simulink library "refrigeration"  (R2014a)
settings: Solver=ode45  StartTime=0.0  StopTime=10.0  RelTol=1e-3
settings Model: Creator=avenger  LastModifiedBy=avenger
settings OptimizationCC: SimCompilerOptimization=off
settings DebuggingCC: MergeDetectMultiDrivingBlocksExec=error  FrameProcessingCompatibilityMsg=error
settings RTWCC: RTWCompilerOptimization=off

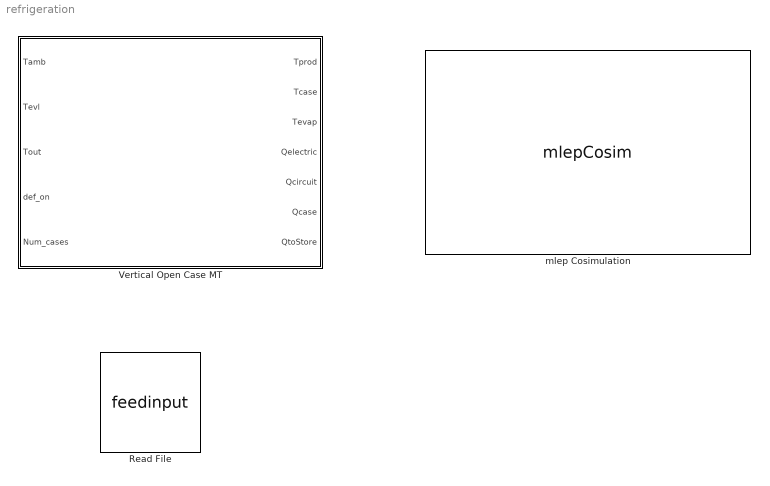
== system refrigeration ==
  Read File : S-Function  FunctionName=feedinput  Parameters=filename,timestep  EnableBusSupport=off  mask(Read Input File){filename='input.txt', timestep=3600}
      mask prompts: filename "File Name:"; timestep "Time Step:"
      mask help:
      | This block reads a file (names passed as parameter) and feeds its input to
      | Simulink at every time step.
  Vertical Open Case MT : Subsystem  AncestorBlock=refrigeration/Vertical Open Case MT
  mlep Cosimulation : S-Function  FunctionName=mlepCosim  Parameters=progname,idf,weather,timeout,step,numinput,numoutput,bcvtbpath  EnableBusSupport=off  mask(S-function: mlepCosim){progname='runenergyplus', idf='supermarket_V810', weather='USA_FL_Miami.Intl.AP.722020_TMY3', timeout=2000, step=300, numinput=1, numoutput=12, bcvtbpath='/home/avenger/Documents/Git/mlep_v2.0/MLE+/bcvtb'}
      mask prompts: progname "E+ Executable:"; idf "IDF File (no .idf extension):"; weather "Weather File (no .epw extension):"; timeout "Timeout (ms):"; step "Sample Time (s):"; numinput "Number of Inputs:"; numoutput "Number of Outputs"; bcvtbpath "Path to bcvtb"
      mask help: This is a S-function block for MLEP.
      mask Display: image('supermarket.png')

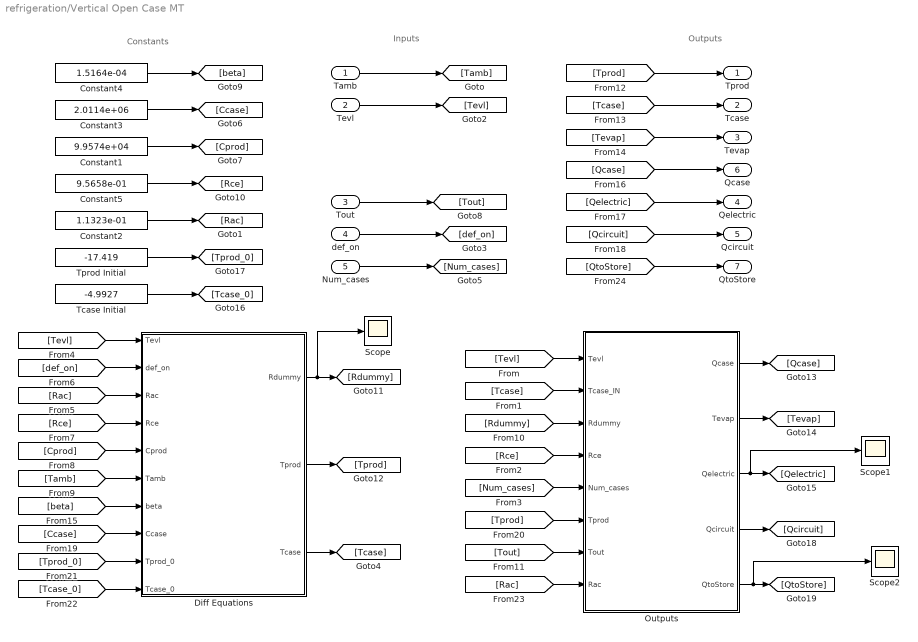
== system refrigeration/Vertical Open Case MT ==
  note: Outputs
  note: Inputs
  note: Constants
  Tamb : Inport
  Tevl : Inport  Port=2
  Tout : Inport  Port=3
  def_on : Inport  Port=4
  Num_cases : Inport  Port=5
  Constant1 : Constant  Value=9.9574e+04
  Constant2 : Constant  Value=1.1323e-01
  Constant3 : Constant  Value=2.0114e+06
  Constant4 : Constant  Value=1.5164e-04
  Constant5 : Constant  Value=9.5658e-01
  Diff Equations : Subsystem
  Outputs : Subsystem
  Scope : Scope
      settings: ShowLegends=on  YMin=-22.5  YMax=32.5
  Scope1 : Scope
      settings: ShowLegends=on  YMin=-22.5  YMax=32.5  SaveName=ScopeData2
  Scope2 : Scope
      settings: ShowLegends=on  YMin=-22.5  YMax=32.5  SaveName=ScopeData7
  Tcase Initial : Constant  Value=-4.9927
  Tprod Initial : Constant  Value=-17.419
  Tprod : Outport
  Tcase : Outport  Port=2
  Tevap : Outport  Port=3
  Qelectric : Outport  Port=4
  Qcircuit : Outport  Port=5
  Qcase : Outport  Port=6
  QtoStore : Outport  Port=7
  wires:
  def_on/1 -> [def_on]
  Num_cases/1 -> [Num_cases]
  Constant3/1 -> [Ccase]
  Constant1/1 -> [Cprod]
  Constant4/1 -> [beta]
  Constant5/1 -> [Rce]
  [Tevl] -> Outputs/1(Tevl)
  [Rce] -> Outputs/4(Rce)
  [Num_cases] -> Outputs/5(Num_cases)
  [Tevl] -> Diff Equations/1(Tevl)
  [Rce] -> Diff Equations/4(Rce)
  [Cprod] -> Diff Equations/5(Cprod)
  [Tamb] -> Diff Equations/6(Tamb)
  Diff Equations/3(Tcase) -> [Tcase]
  Diff Equations/1(Rdummy) -> Scope/1, [Rdummy]
  Diff Equations/2(Tprod) -> [Tprod]
  [Tcase] -> Outputs/2(Tcase_IN)
  [Rdummy] -> Outputs/3(Rdummy)
  [Qelectric] -> Qelectric/1
  [Qcircuit] -> Qcircuit/1
  [Qcase] -> Qcase/1
  Outputs/3(Qelectric) -> Scope1/1, [Qelectric]
  Outputs/1(Qcase) -> [Qcase]
  Outputs/2(Tevap) -> [Tevap]
  Outputs/4(Qcircuit) -> [Qcircuit]
  [beta] -> Diff Equations/7(beta)
  [Ccase] -> Diff Equations/8(Ccase)
  [Tprod] -> Outputs/6(Tprod)
  Tprod Initial/1 -> [Tprod_0]
  Tcase Initial/1 -> [Tcase_0]
  Tamb/1 -> [Tamb]
  Tevl/1 -> [Tevl]
  [Tprod] -> Tprod/1
  [Tcase] -> Tcase/1
  [Tevap] -> Tevap/1
  [Rac] -> Diff Equations/3(Rac)
  [def_on] -> Diff Equations/2(def_on)
  Constant2/1 -> [Rac]
  [Tprod_0] -> Diff Equations/9(Tprod_0)
  [Tcase_0] -> Diff Equations/10(Tcase_0)
  Tout/1 -> [Tout]
  [Tout] -> Outputs/7(Tout)
  [Rac] -> Outputs/8(Rac)
  Outputs/5(QtoStore) -> Scope2/1, [QtoStore]
  [QtoStore] -> QtoStore/1

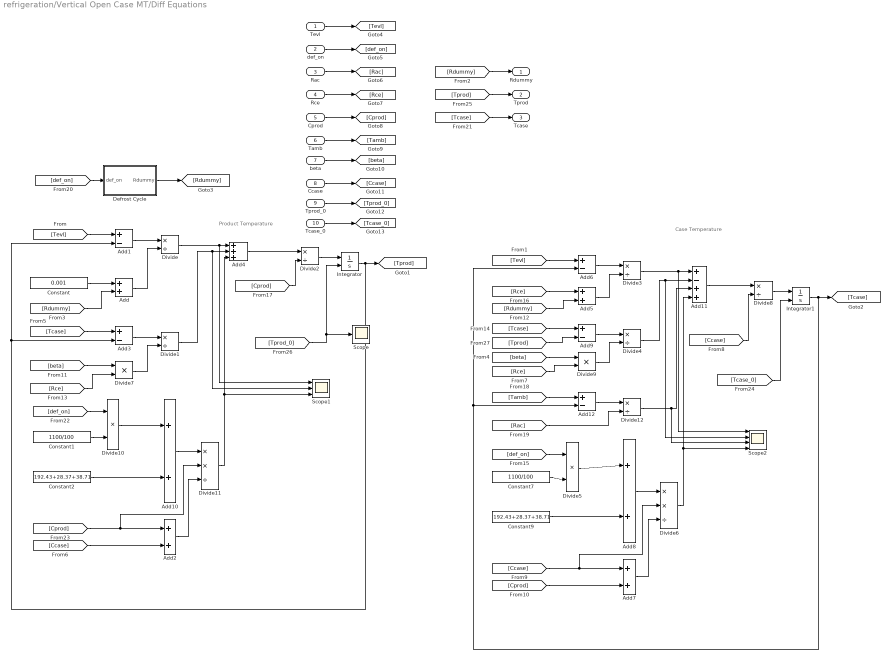
== system refrigeration/Vertical Open Case MT/Diff Equations ==
  note: Product Temperature
  note: Case Temperature
  Tevl : Inport
  def_on : Inport  Port=2
  Rac : Inport  Port=3
  Rce : Inport  Port=4
  Cprod : Inport  Port=5
  Tamb : Inport  Port=6
  beta : Inport  Port=7
  Ccase : Inport  Port=8
  Tprod_0 : Inport  Port=9
  Tcase_0 : Inport  Port=10
  Add{,2,5,7..8,10} (6 alike) : Sum
  Add{1,3,6,9,12} (5 alike) : Sum  Inputs=+-
  Add11 : Sum  Inputs=+-++
  Add4 : Sum  Inputs=+++
  Constant : Constant  Value=0.001
  Constant1 : Constant  Value=1100/100
  Constant2 : Constant  Value=192.43+28.37+38.71
  Constant7 : Constant  Value=1100/100
  Constant9 : Constant  Value=192.43+28.37+38.71
  Defrost Cycle : Subsystem  TreatAsAtomicUnit=on
  Divide{,1..4,8,12} (7 alike) : Product  Inputs=*/
  Divide{5,7,9..10} (4 alike) : Product  Inputs=**
  Divide11 : Product  Inputs=**/
  Divide6 : Product  Inputs=**/
  Integrator : Integrator  InitialConditionSource=external
  Integrator1 : Integrator  InitialConditionSource=external
  Scope : Scope
      settings: ShowLegends=on  YMin=-22.5  YMax=32.5
  Scope1 : Scope  NumInputPorts=3
      settings: ShowLegends=on  YMin=-47500~20000~12.241  YMax=-20000~47500~12.241  SaveName=ScopeData2
  Scope2 : Scope  NumInputPorts=4
      settings: ShowLegends=on  YMin=-62.5~-1~-180~247.269  YMax=-45~1~-30~247.269  SaveName=ScopeData3
  Rdummy : Outport
  Tprod : Outport  Port=2
  Tcase : Outport  Port=3
  wires:
  [Tprod] -> Add9/2
  Divide3/1 -> Add11/1, Scope2/1
  Constant/1 -> Add/1
  [Rdummy] -> Add/2
  [Tevl] -> Add1/1
  Add1/1 -> Divide/1
  Add/1 -> Divide/2
  [Tcase] -> Add3/1
  Integrator/1 -> Add3/2, Add1/2, [Tprod]
  Add3/1 -> Divide1/1
  Divide7/1 -> Divide1/2
  Divide/1 -> Add4/1, Scope1/1
  Divide1/1 -> Add4/2, Scope1/2
  Add4/1 -> Divide2/1
  Divide2/1 -> Integrator/1
  [beta] -> Divide7/1
  [Rce] -> Divide7/2
  [Cprod] -> Divide2/2
  [def_on] -> Defrost Cycle/1(def_on)
  Defrost Cycle/1(Rdummy) -> [Rdummy]
  Tevl/1 -> [Tevl]
  def_on/1 -> [def_on]
  Rac/1 -> [Rac]
  Rce/1 -> [Rce]
  Cprod/1 -> [Cprod]
  Tamb/1 -> [Tamb]
  [Rdummy] -> Rdummy/1
  [Tprod] -> Tprod/1
  [Tcase] -> Tcase/1
  beta/1 -> [beta]
  Ccase/1 -> [Ccase]
  [Rce] -> Add5/1
  [Rdummy] -> Add5/2
  [Tevl] -> Add6/1
  Add6/1 -> Divide3/1
  Add5/1 -> Divide3/2
  [Tcase] -> Add9/1
  Add9/1 -> Divide4/1
  Divide9/1 -> Divide4/2
  Divide4/1 -> Add11/2, Scope2/2
  Add11/1 -> Divide8/1
  Divide8/1 -> Integrator1/1
  [beta] -> Divide9/1
  [Rce] -> Divide9/2
  [Ccase] -> Divide8/2
  [def_on] -> Divide5/1
  Constant7/1 -> Divide5/2
  Divide5/1 -> Add8/1
  Constant9/1 -> Add8/2
  Add8/1 -> Divide6/1
  [Ccase] -> Add7/1, Divide6/2
  [Cprod] -> Add7/2
  Add7/1 -> Divide6/3
  [Tamb] -> Add12/1
  Integrator1/1 -> [Tcase], Add12/2, Add6/2
  Add12/1 -> Divide12/1
  [Rac] -> Divide12/2
  Divide12/1 -> Add11/3, Scope2/3
  Divide6/1 -> Add11/4, Scope2/4
  [def_on] -> Divide10/1
  Constant1/1 -> Divide10/2
  Divide10/1 -> Add10/1
  Constant2/1 -> Add10/2
  Add10/1 -> Divide11/1
  [Cprod] -> Add2/1, Divide11/2
  [Ccase] -> Add2/2
  Add2/1 -> Divide11/3
  Divide11/1 -> Add4/3, Scope1/3
  [Tcase_0] -> Integrator1/2
  [Tprod_0] -> Integrator/2, Scope/1
  Tprod_0/1 -> [Tprod_0]
  Tcase_0/1 -> [Tcase_0]

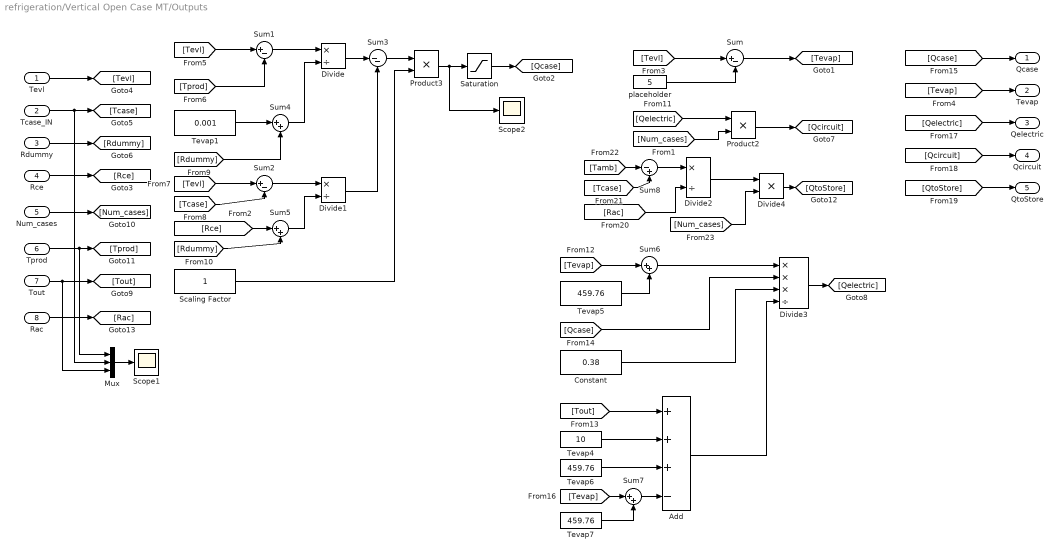
== system refrigeration/Vertical Open Case MT/Outputs ==
  Tevl : Inport
  Tcase_IN : Inport  Port=2
  Rdummy : Inport  Port=3
  Rce : Inport  Port=4
  Num_cases : Inport  Port=5
  Tprod : Inport  Port=6
  Tout : Inport  Port=7
  Rac : Inport  Port=8
  Add : Sum  Inputs=+++-
  Constant : Constant  Value=0.38
  Divide : Product  Inputs=*/
  Divide1 : Product  Inputs=*/
  Divide2 : Product  Inputs=*/
  Divide3 : Product  Inputs=***/
  Divide4 : Product  Inputs=**
  Mux : Mux  Inputs=3
  Product2 : Product
  Product3 : Product
  Saturation : Saturate  UpperLimit=Inf
  Scaling Factor : Constant
  Scope1 : Scope
      settings: ShowLegends=on  YMin=-22.5  YMax=32.5  SaveName=ScopeData3
  Scope2 : Scope
      settings: ShowLegends=on  YMin=-22.5  YMax=32.5  SaveName=ScopeData6
  Sum : Sum  Inputs=|+-
  Sum1 : Sum  Inputs=|+-
  Sum2 : Sum  Inputs=|+-
  Sum3 : Sum  Inputs=|--
  Sum{4..7} (4 alike) : Sum  Inputs=|++
  Sum8 : Sum  Inputs=|-+
  Tevap1 : Constant  Value=0.001
  Tevap4 : Constant  Value=10
  Tevap5 : Constant  Value=459.76
  Tevap6 : Constant  Value=459.76
  Tevap7 : Constant  Value=459.76
  placeholder : Constant  Value=5
  Qcase : Outport
  Tevap : Outport  Port=2
  Qelectric : Outport  Port=3
  Qcircuit : Outport  Port=4
  QtoStore : Outport  Port=5
  wires:
  [Tevl] -> Sum/1
  Sum/1 -> [Tevap]
  placeholder/1 -> Sum/2
  [Tevl] -> Sum1/1
  [Tprod] -> Sum1/2
  [Tevl] -> Sum2/1
  [Tcase] -> Sum2/2
  Sum1/1 -> Divide/1
  Tevap1/1 -> Sum4/1
  [Rdummy] -> Sum4/2
  Sum4/1 -> Divide/2
  Sum2/1 -> Divide1/1
  [Rce] -> Sum5/1
  [Rdummy] -> Sum5/2
  Sum5/1 -> Divide1/2
  Divide/1 -> Sum3/1
  Divide1/1 -> Sum3/2
  [Tevap] -> Sum6/1
  Tevap5/1 -> Sum6/2
  Sum6/1 -> Divide3/1
  Divide3/1 -> [Qelectric]
  [Qcase] -> Divide3/2
  Constant/1 -> Divide3/3
  [Qelectric] -> Product2/1
  [Num_cases] -> Product2/2
  Sum3/1 -> Product3/1
  Scaling Factor/1 -> Product3/2
  Product2/1 -> [Qcircuit]
  [Qcase] -> Qcase/1
  [Tevap] -> Tevap/1
  [Qelectric] -> Qelectric/1
  [Qcircuit] -> Qcircuit/1
  Tevl/1 -> [Tevl]
  Tcase_IN/1 -> Mux/2, [Tcase]
  Rdummy/1 -> [Rdummy]
  Rce/1 -> [Rce]
  Num_cases/1 -> [Num_cases]
  Tout/1 -> Mux/3, [Tout]
  Add/1 -> Divide3/4
  [Tout] -> Add/1
  Tevap4/1 -> Add/2
  Tevap6/1 -> Add/3
  [Tevap] -> Sum7/1
  Sum7/1 -> Add/4
  Tevap7/1 -> Sum7/2
  Mux/1 -> Scope1/1
  Tprod/1 -> Mux/1, [Tprod]
  Product3/1 -> Scope2/1, Saturation/1
  [QtoStore] -> QtoStore/1
  Divide2/1 -> Divide4/1
  [Tamb] -> Sum8/1
  [Tcase] -> Sum8/2
  Sum8/1 -> Divide2/1
  [Rac] -> Divide2/2
  Rac/1 -> [Rac]
  Saturation/1 -> [Qcase]
  Divide4/1 -> [QtoStore]
  [Num_cases] -> Divide4/2

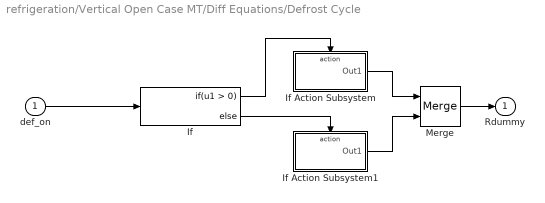
== system refrigeration/Vertical Open Case MT/Diff Equations/Defrost Cycle ==
  def_on : Inport
  If : If
  If Action Subsystem : Subsystem  TreatAsAtomicUnit=on
  If Action Subsystem1 : Subsystem  TreatAsAtomicUnit=on
  Merge : Merge
  Rdummy : Outport
  wires:
  def_on/1 -> If/1
  If/2 -> If Action Subsystem1/Action
  If/1 -> If Action Subsystem/Action
  If Action Subsystem/1(Out1) -> Merge/1
  If Action Subsystem1/1(Out1) -> Merge/2
  Merge/1 -> Rdummy/1

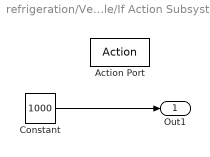
== system refrigeration/Vertical Open Case MT/Diff Equations/Defrost Cycle/If Action Subsystem ==
  Action Port : ActionPort
  Constant : Constant  Value=1000
  Out1 : Outport
  wires:
  Constant/1 -> Out1/1

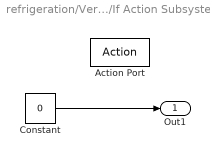
== system refrigeration/Vertical Open Case MT/Diff Equations/Defrost Cycle/If Action Subsystem1 ==
  Action Port : ActionPort
  Constant : Constant  Value=0
  Out1 : Outport
  wires:
  Constant/1 -> Out1/1
